simulink model "honors_drone_4b"  (R2017a)
settings: Solver=FixedStepAuto  StartTime=0.0  StopTime=10.0  FixedStep=0.04  RelTol=1e-3
values from neighbouring files (symbols this model uses):
  g = 9.81    [run_file.m]
  m = 0.429    [run_file.m]
settings Model: Creator=s154530  LastModifiedBy=s166315
settings DataIOCC: SaveFormat=Array

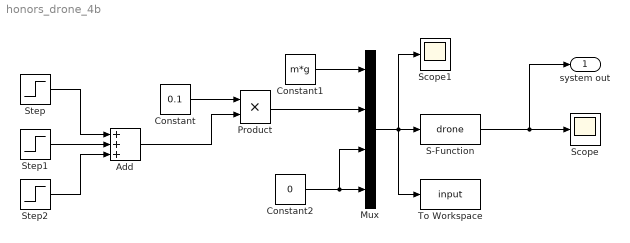
== system honors_drone_4b ==
  Add : Sum  Inputs=+++
  Constant : Constant  Value=0.1
  Constant1 : Constant  Value=m*g
  Constant2 : Constant  Value=0
  Mux : Mux
  Product : Product
  S-Function : S-Function  FunctionName=drone  Parameters=x0, m, g, Ix, Iy, Iz  SFunctionDeploymentMode=off  EnableBusSupport=off
  Scope : Scope
  Scope1 : Scope
  Step : Step  SampleTime=0
  Step1 : Step  Time=1.1  After=-2  SampleTime=0
  Step2 : Step  Time=1.2  SampleTime=0
  To Workspace : ToWorkspace  VariableName=input  SaveFormat=Timeseries  SampleTime=-1
      settings: MaxDataPoints=Inf
  system out : Outport
  wires:
  S-Function/1 -> system out/1, Scope/1
  Step/1 -> Add/1
  Step1/1 -> Add/2
  Step2/1 -> Add/3
  Add/1 -> Product/2
  Constant/1 -> Product/1
  Mux/1 -> To Workspace/1, Scope1/1, S-Function/1
  Constant2/1 -> Mux/3, Mux/4
  Constant1/1 -> Mux/1
  Product/1 -> Mux/2
